simulink model "autopilot_vtolsim"  (R2019a)
settings: Solver=ode15s  StartTime=0.0  StopTime=10000  RelTol=1e-3  EnableMultiTasking=on
InitFcn:
  | clear all
  | path(pathdef)
  | addpath('.')
  | simulation_parameters
  | wind_parameters
  | vtol_parameters
StartFcn:
  | clear all
  | path(pathdef)
  | addpath('.')
  | simulation_parameters
  | wind_parameters
  | vtol_parameters
undefined symbols (not defined in the file or in its folder): AP, autopilot, drawAircraft, forces_moments, init_states, plane_states, plotvtolstatevariables, SIM, true_states, vtol, vtol_dynamics, WIND
libraries: simulink x3
settings Model: Creator=beard  LastModifiedBy=VTOL_HYD
settings DataIOCC: LimitDataPoints=on  SaveFormat=Array  SignalLoggingSaveFormat=ModelDataLogs  ReturnWorkspaceOutputs=off
settings OptimizationCC: ExpressionDepthLimit=2147483647  InitFltsAndDblsToZero=on  LifeSpan=inf
settings DebuggingCC: UnderspecifiedInitializationDetection=Classic  MergeDetectMultiDrivingBlocksExec=none  FcnCallInpInsideContextMsg=warning  AllowSymbolicDim=off  StateNameClashWarn=warning  PregeneratedLibrarySubsystemCodeDiagnostic=none  SFUnexpectedBacktrackingDiag=warning  SFNoUnconditionalDefaultTransitionDiag=warning  SFExecutionAtInitializationDiag=none  ArithmeticOperatorsInVariantConditions=warning
settings HardwareCC: ProdBitPerPointer=32  ProdBitPerSizeT=32  ProdBitPerPtrDiffT=32  ProdLargestAtomicFloat=None  ProdIntDivRoundTo=Undefined  ProdEndianess=Unspecified  ProdWordSize=32  ProdHWDeviceType=32-bit Generic
settings ModelReferenceCC: PropagateSignalLabelsOutOfModel=off
settings SFSimCC: SimUseLocalCustomCode=off
settings RTWCC: RTWUseLocalCustomCode=off
settings CodeAppCC: StateflowObjectComments=on
settings GRTTargetCC: TargetLangStandard=C89/C90 (ANSI)  GeneratePreprocessorConditionals=Disable all  CombineOutputUpdateFcns=off  GRTInterface=on
settings ConfigComp: CovMetricSettings=dw  CovHtmlReporting=on  CovSaveCumulativeToWorkspaceVar=on  CovSaveSingleToWorkspaceVar=on  CovExternalEMLEnable=off  CovSFcnEnable=off

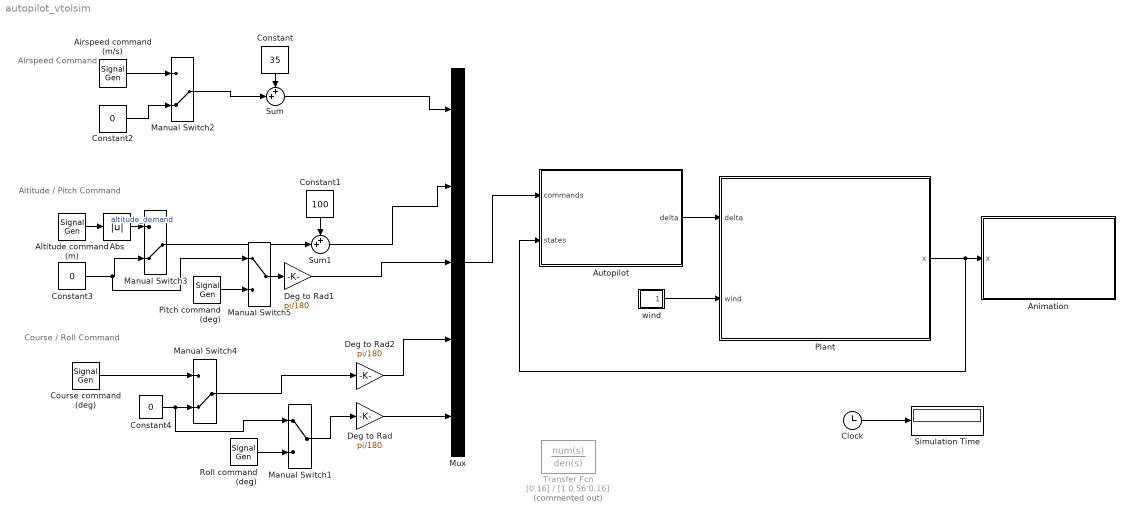
== system autopilot_vtolsim ==
  note: Airspeed Command
  note: Altitude / Pitch Command
  note: Course / Roll Command
  Abs : Abs
  Airspeed command (m/s) : SignalGenerator  WaveForm=square  Amplitude=5  Frequency=0.012
  Altitude command (m) : SignalGenerator  Amplitude=15  Frequency=.02
  Animation : Subsystem
      mask Display: image(imread('animation.jpg'))
  Autopilot : Subsystem
      mask Display: image(imread('stm32.jpg'))
  Clock : Clock
  Constant : Constant  Value=35
  Constant1 : Constant  Value=100
  Constant2 : Constant  Value=0
  Constant3 : Constant  Value=0
  Constant4 : Constant  Value=0
  Course command (deg) : SignalGenerator  Amplitude=45  Frequency=.012
  Deg to Rad : Gain  Gain=pi/180
  Deg to Rad1 : Gain  Gain=pi/180
  Deg to Rad2 : Gain  Gain=pi/180
  Manual Switch1 : ManualSwitch
  Manual Switch2 : ManualSwitch  CurrentSetting=0
  Manual Switch3 : ManualSwitch  CurrentSetting=0
  Manual Switch4 : ManualSwitch  CurrentSetting=0
  Manual Switch5 : ManualSwitch
  Mux : Mux  Inputs=5
  Pitch command (deg) : SignalGenerator  Amplitude=20  Frequency=0.1
  Plant : Subsystem
      mask Display: image(imread('vtol.jpeg'))
  Roll command (deg) : SignalGenerator  WaveForm=square  Amplitude=45  Frequency=.1
  Simulation Time : Display
  Sum : Sum  Inputs=++|
  Sum1 : Sum  Inputs=++|
  Transfer Fcn : TransferFcn  Commented=on  Numerator=[0.16]  Denominator=[1 0.56 0.16]
  wind : Subsystem
  wires:
  Clock/1 -> Simulation Time/1
  wind/1(Wind) -> Plant/2(wind)
  Plant/1(x) -> Autopilot/2(states), Animation/1(x)
  Autopilot/1(delta) -> Plant/1(delta)
  Deg to Rad/1 -> Mux/5
  Sum/1 -> Mux/1
  Constant/1 -> Sum/1
  Sum1/1 -> Mux/2
  Constant1/1 -> Sum1/1
  Deg to Rad1/1 -> Mux/3
  Airspeed command (m/s)/1 -> Manual Switch2/1
  Constant2/1 -> Manual Switch2/2
  Manual Switch3/1 -> Sum1/2
  Constant3/1 -> Manual Switch5/1, Manual Switch3/2
  Constant4/1 -> Manual Switch1/1, Manual Switch4/2
  Manual Switch4/1 -> Deg to Rad2/1
  Course command (deg)/1 -> Manual Switch4/1
  Manual Switch2/1 -> Sum/2
  Deg to Rad2/1 -> Mux/4
  Mux/1 -> Autopilot/1(commands)
  Roll command (deg)/1 -> Manual Switch1/2
  Manual Switch1/1 -> Deg to Rad/1
  Manual Switch5/1 -> Deg to Rad1/1
  Pitch command (deg)/1 -> Manual Switch5/2
  Altitude command (m)/1 -> Abs/1
  Abs/1 -> Manual Switch3/1  "altitude_demand"

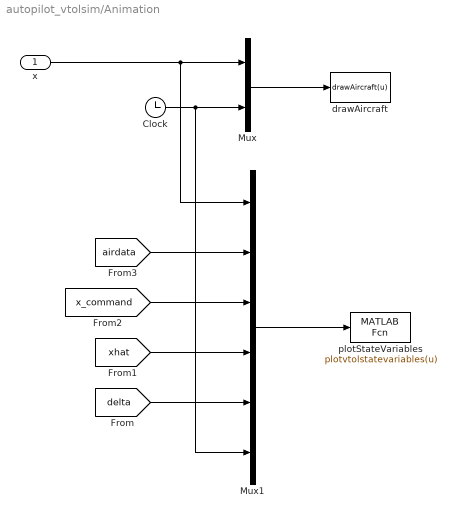
== system autopilot_vtolsim/Animation ==
  x : Inport
  Clock : Clock
  Mux : Mux  Inputs=2
  Mux1 : Mux  Inputs=6
  drawAircraft : MATLABFcn  MATLABFcn=drawAircraft(u)  OutputDimensions=0
  plotStateVariables : MATLABFcn  MATLABFcn=plotvtolstatevariables(u)  OutputDimensions=0
  wires:
  Mux/1 -> drawAircraft/1
  x/1 -> Mux/1, Mux1/1
  Clock/1 -> Mux/2, Mux1/6
  Mux1/1 -> plotStateVariables/1
  [xhat] -> Mux1/4
  [x_command] -> Mux1/3
  [delta] -> Mux1/5
  [airdata] -> Mux1/2

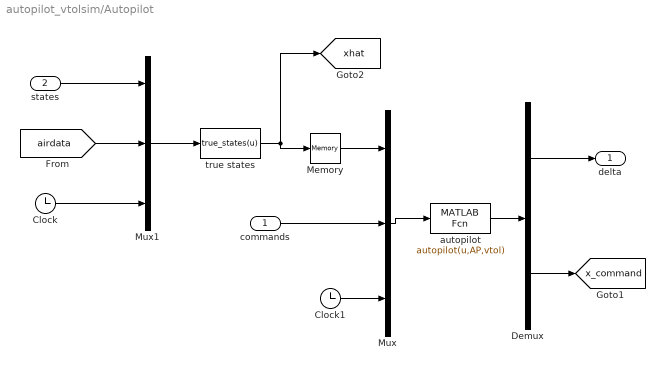
== system autopilot_vtolsim/Autopilot ==
  commands : Inport
  states : Inport  Port=2
  Clock : Clock
  Clock1 : Clock
  Demux : Demux  Outputs=[4;12]
  Memory : Memory  InheritSampleTime=on  LinearizeAsDelay=on
  Mux : Mux  Inputs=3
  Mux1 : Mux  Inputs=3
  autopilot : MATLABFcn  MATLABFcn=autopilot(u,AP,vtol)  OutputDimensions=4+12
  true states : MATLABFcn  MATLABFcn=true_states(u)  OutputDimensions=19
  delta : Outport
  tag scope: x_command=global, xhat=global
  wires:
  Mux/1 -> autopilot/1
  Clock/1 -> Mux1/3
  autopilot/1 -> Demux/1
  Demux/1 -> delta/1
  Demux/2 -> [x_command]
  commands/1 -> Mux/2
  Mux1/1 -> true states/1
  states/1 -> Mux1/1
  true states/1 -> [xhat], Memory/1
  [airdata] -> Mux1/2
  Memory/1 -> Mux/1
  Clock1/1 -> Mux/3

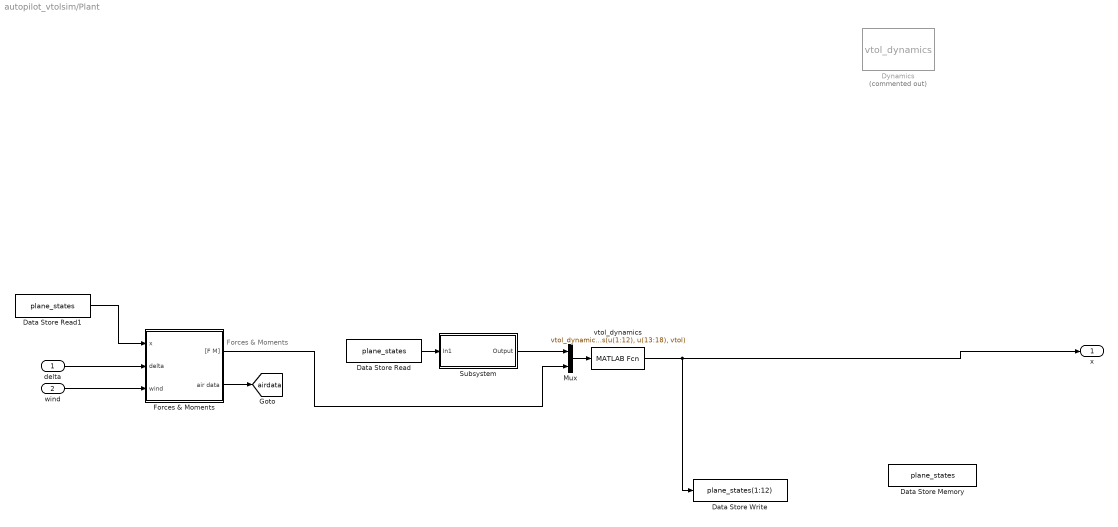
== system autopilot_vtolsim/Plant ==
  note: Forces & Moments
  delta : Inport
  wind : Inport  Port=2
  Data Store Memory : DataStoreMemory  DataStoreName=plane_states  ReadBeforeWriteMsg=warning  WriteAfterWriteMsg=warning  WriteAfterReadMsg=warning  InitialValue=[0;0;0;0;0;0;0;0;0;0;0;0]  ShowAdditionalParam=off
  Data Store Read : DataStoreRead  DataStoreName=plane_states
  Data Store Read1 : DataStoreRead  DataStoreName=plane_states
  Data Store Write : DataStoreWrite  DataStoreName=plane_states  DataStoreElements=plane_states(1:12)
  Dynamics : S-Function  Commented=on  InitFcn=|  FunctionName=vtol_dynamics  Parameters=vtol  SFunctionDeploymentMode=off  EnableBusSupport=off
      | addpath('.')
      | simulation_parameters
      | vtol_parameters
  Forces & Moments : Subsystem
  Mux : Mux  Inputs=2
  Subsystem : Subsystem  InitFcn=|
      | clear all
      | path(pathdef)
      | addpath('.')
  vtol_dynamics : MATLABFcn  MATLABFcn=vtol_dynamics(u(1:12), u(13:18), vtol)  OutputDimensions=12
  x : Outport
  tag scope: airdata=global
  wires:
  vtol_dynamics/1 -> x/1, Data Store Write/1
  Forces & Moments/2(air data) -> [airdata]
  delta/1 -> Forces & Moments/2(delta)
  wind/1 -> Forces & Moments/3(wind)
  Data Store Read/1 -> Subsystem/1(In1)
  Forces & Moments/1("[F M]") -> Mux/2
  Mux/1 -> vtol_dynamics/1
  Subsystem/1(Output) -> Mux/1
  Data Store Read1/1 -> Forces & Moments/1(x)

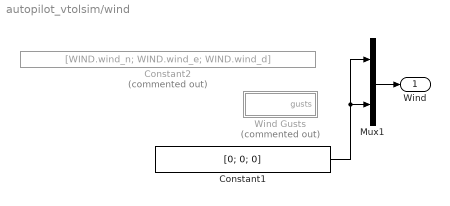
== system autopilot_vtolsim/wind ==
  Constant1 : Constant  Value=[0; 0; 0]
  Constant2 : Constant  Commented=on  Value=[WIND.wind_n; WIND.wind_e; WIND.wind_d]
  Mux1 : Mux  Inputs=2
  Wind Gusts : Subsystem  Commented=on
  Wind : Outport
  wires:
  Mux1/1 -> Wind/1
  Constant1/1 -> Mux1/2, Mux1/1

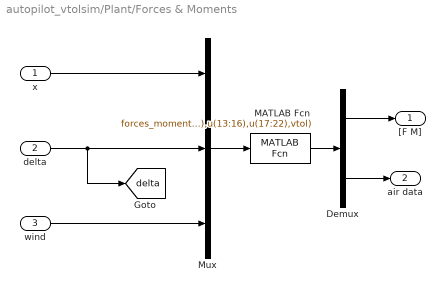
== system autopilot_vtolsim/Plant/Forces & Moments ==
  x : Inport
  delta : Inport  Port=2
  wind : Inport  Port=3
  Demux : Demux  Outputs=[6;6]
  MATLAB Fcn : MATLABFcn  MATLABFcn=forces_moments(u(1:12),u(13:16),u(17:22),vtol)  OutputDimensions=12
  Mux : Mux  Inputs=3
  "[F M]" : Outport
  air data : Outport  Port=2
  tag scope: delta=global
  wires:
  Demux/2 -> air data/1
  Mux/1 -> MATLAB Fcn/1
  Demux/1 -> "[F M]"/1
  MATLAB Fcn/1 -> Demux/1
  wind/1 -> Mux/3
  delta/1 -> Mux/2, [delta]
  x/1 -> Mux/1

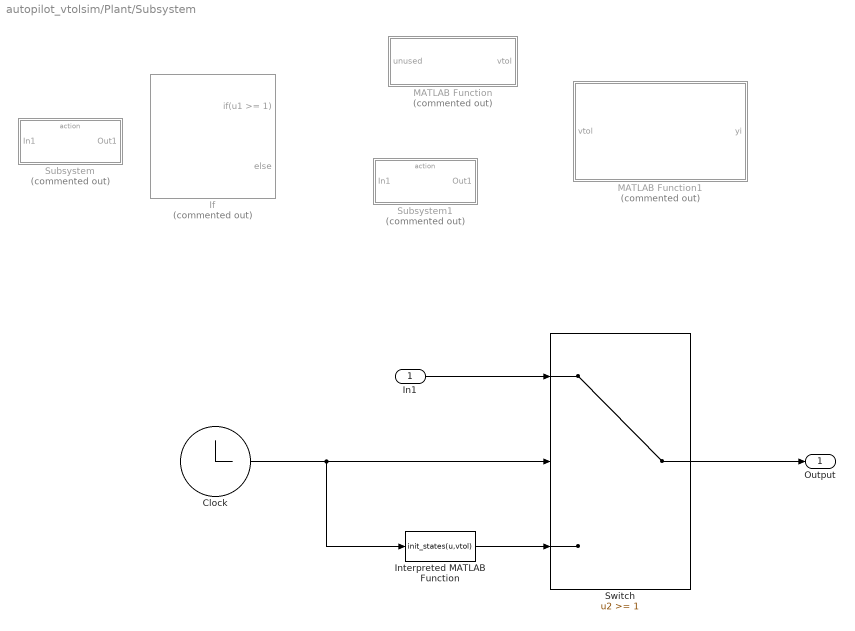
== system autopilot_vtolsim/Plant/Subsystem ==
  In1 : Inport
  Clock : Clock
  If : If  Commented=on  IfExpression=u1 >= 1
  Interpreted MATLAB Function : MATLABFcn  MATLABFcn=init_states(u,vtol)  OutputDimensions=12
  MATLAB Function : MATLAB Function  Commented=on  TreatAsAtomicUnit=on
  MATLAB Function1 : MATLAB Function  Commented=on  InitFcn=|  TreatAsAtomicUnit=on
      | path(pathdef)
      | addpath('.')
  Subsystem : Subsystem  Commented=on
  Subsystem1 : Subsystem  Commented=on
  Switch : Switch  Threshold=1  ZeroCross=off
  Output : Outport
  wires:
  Switch/1 -> Output/1
  In1/1 -> Switch/1
  Interpreted MATLAB Function/1 -> Switch/3
  Clock/1 -> Interpreted MATLAB Function/1, Switch/2

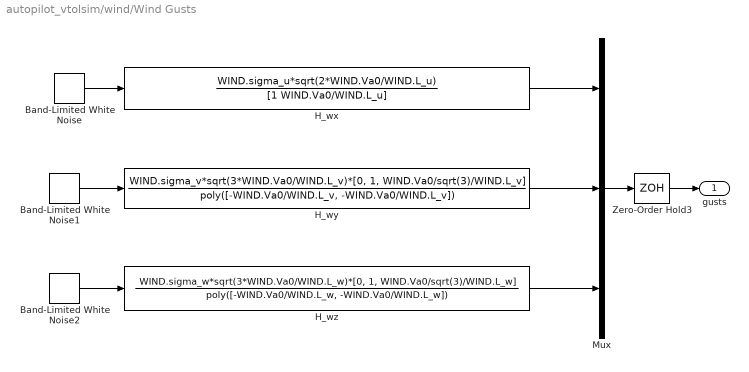
== system autopilot_vtolsim/wind/Wind Gusts ==
  Band-Limited White Noise : simulink/Sources/Band-Limited White Noise  Cov=[1]  Ts=SIM.ts_simulation  seed=[23341]
  Band-Limited White Noise1 : simulink/Sources/Band-Limited White Noise  Cov=[1]  Ts=SIM.ts_simulation  seed=[23341]
  Band-Limited White Noise2 : simulink/Sources/Band-Limited White Noise  Cov=[1]  Ts=SIM.ts_simulation  seed=[23341]
  H_wx : TransferFcn  Numerator=WIND.sigma_u*sqrt(2*WIND.Va0/WIND.L_u)  Denominator=[1 WIND.Va0/WIND.L_u]
  H_wy : TransferFcn  Numerator=WIND.sigma_v*sqrt(3*WIND.Va0/WIND.L_v)*[0, 1, WIND.Va0/sqrt(3)/WIND.L_v]  Denominator=poly([-WIND.Va0/WIND.L_v, -WIND.Va0/WIND.L_v])
  H_wz : TransferFcn  Numerator=WIND.sigma_w*sqrt(3*WIND.Va0/WIND.L_w)*[0, 1, WIND.Va0/sqrt(3)/WIND.L_w]  Denominator=poly([-WIND.Va0/WIND.L_w, -WIND.Va0/WIND.L_w])
  Mux : Mux  Inputs=3
  Zero-Order Hold3 : ZeroOrderHold  SampleTime=SIM.ts_simulation
  gusts : Outport
  wires:
  H_wx/1 -> Mux/1
  Band-Limited White Noise/1 -> H_wx/1
  H_wy/1 -> Mux/2
  Band-Limited White Noise1/1 -> H_wy/1
  H_wz/1 -> Mux/3
  Band-Limited White Noise2/1 -> H_wz/1
  Mux/1 -> Zero-Order Hold3/1
  Zero-Order Hold3/1 -> gusts/1

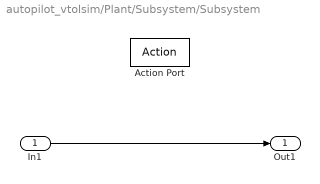
== system autopilot_vtolsim/Plant/Subsystem/Subsystem ==
  In1 : Inport
  Action Port : ActionPort  InitializeStates=reset
  Out1 : Outport
  wires:
  In1/1 -> Out1/1

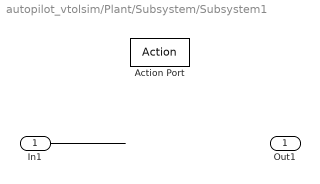
== system autopilot_vtolsim/Plant/Subsystem/Subsystem1 ==
  In1 : Inport
  Action Port : ActionPort  InitializeStates=reset
  Out1 : Outport
  wires:
  In1/1 -> ?
  ? -> Out1/1

== matlab function autopilot_vtolsim/Plant/Subsystem/MATLAB Function1 ==
  data: yi output; vtol input
function yi = init_states(vtol)
   yi = vtol;
end

== matlab function autopilot_vtolsim/Plant/Subsystem/MATLAB Function ==
  data: vtol output double; unused input
% initialize the VTOL viewer
function vtol = vtol_parameters(~)

    vtol.pn0    = 0;     % initial North position
	vtol.pe0    = 0;     % initial East position
	vtol.pd0    = 0;  % initial Down position (negative altitude)
	vtol.u0     = 0;     % initial velocity along body x-axis
	vtol.v0     = 0;     % initial velocity along body y-axis
	vtol.w0     = 0;     % initial velocity along body z-axis
	vtol.phi0   = 0;     % initial roll angle
	vtol.theta0 = 0;     % initial pitch angle
	vtol.psi0   = 0;     % initial yaw angle
% 	e = Euler2Quaternion(vtol.phi0,vtol.theta0,vtol.psi0);
% 	vtol.e0     = e(1);  % initial quaternion
% 	vtol.e1     = e(2);
% 	vtol.e2     = e(3);
% 	vtol.e3     = e(4);
	vtol.p0     = 0;     % initial body frame roll rate
	vtol.q0     = 0;     % initial body frame pitch rate
	vtol.r0     = 0;     % initial body frame yaw rate
    
	%physical parameters of airframe
	vtol.gravity = 9.81;
	vtol.mass = 13.5;
	vtol.Jx   = 0.8244;
	vtol.Jy   = 1.135;
	vtol.Jz   = 1.759;
	vtol.Jxz  = 0.1204;
	vtol.S_wing        = 0.55;
	vtol.b             = 2.90;
	vtol.c             = 0.19;
	vtol.S_prop        = 0.2027;
	vtol.rho           = 1.2682;
	vtol.e             = 0.9;
	vtol.AR            = vtol.b^2/vtol.S_wing;

	% Gamma parameters 
	vtol.Gamma  = vtol.Jx*vtol.Jz-vtol.Jxz^2;
	vtol.Gamma1 = (vtol.Jxz*(vtol.Jx-vtol.Jy+vtol.Jz))/vtol.Gamma;
	vtol.Gamma2 = (vtol.Jz*(vtol.Jz-vtol.Jy)+vtol.Jxz*vtol.Jxz)/vtol.Gamma;
	vtol.Gamma3 = vtol.Jz/vtol.Gamma;
	vtol.Gamma4 = vtol.Jxz/vtol.Gamma;
	vtol.Gamma5 = (vtol.Jz-vtol.Jx)/vtol.Jy;
	vtol.Gamma6 = vtol.Jxz/vtol.Jy;
	vtol.Gamma7 = (vtol.Jx*(vtol.Jx-vtol.Jy)+vtol.Jxz*vtol.Jxz)/vtol.Gamma;
	vtol.Gamma8 = vtol.Jx/vtol.Gamma;

	%%%%%%%%%%%%%%%%%%%%%%%%%%%%%%%%%
	% aerodynamic coefficients
	vtol.C_L_0         = 0.28;
	vtol.C_D_0         = 0.03;
	vtol.C_m_0         = -0.02338;
	vtol.C_L_alpha     = 3.45;
	vtol.C_D_alpha     = 0.30;
	vtol.C_m_alpha     = -0.38;
	vtol.C_L_q         = 0;
	vtol.C_D_q         = 0.0;
	vtol.C_m_q         = -3.6;
	vtol.C_L_delta_e   = -0.36;
	vtol.C_D_delta_e   = 0.0;
	vtol.C_m_delta_e   = -0.5;
	vtol.M             = 50;
	vtol.alpha0        = 0.4712;
	vtol.epsilon       = 0.16;
	vtol.C_D_p         = 0.0437;

	vtol.C_Y_0         = 0.0;
	vtol.C_ell_0       = 0.0;
	vtol.C_n_0         = 0.0;
	vtol.C_Y_beta      = -0.98;
	vtol.C_ell_beta    = -0.12;
	vtol.C_n_beta      = 0.25;
	vtol.C_Y_p         = 0.0;
	vtol.C_ell_p       = -0.26;
	vtol.C_n_p         = 0.022;
	vtol.C_Y_r         = 0.0;
	vtol.C_ell_r       = 0.14;
	vtol.C_n_r         = -0.35;
	vtol.C_Y_delta_a   = 0.0;
	vtol.C_ell_delta_a = 0.08;
	vtol.C_n_delta_a   = 0.06;
	vtol.C_Y_delta_r   = -0.17;
	vtol.C_ell_delta_r = 0.105;
	vtol.C_n_delta_r   = -0.032;

	% Parameters for propulsion thrust and torque models
	vtol.D_prop = 0.508;     % prop diameter in m

	% Motor parameters
	vtol.K_V = 145;                    % from datasheet RPM/V
	vtol.KQ = (1/vtol.K_V)*60/(2*pi);   % KQ in N-m/A, V-s/rad
	vtol.R_motor = 0.042;              % ohms
	vtol.i0 = 1.5;                     % no-load (zero-torque) current (A)

	% Inputs
	vtol.ncells = 12;
	vtol.V_max = 3.7*vtol.ncells;       % max voltage for specified number of battery cells

	% Coeffiecients from prop_data fit
	vtol.C_Q2 = -0.01664;
	vtol.C_Q1 = 0.004970;
	vtol.C_Q0 = 0.005230;

	vtol.C_T2 = -0.1079;
	vtol.C_T1 = -0.06044;
	vtol.C_T0 = 0.09357;

end
